simulink model "BalanceSimulink"  (R2023b)
settings: Solver=ode14x  StartTime=0.0  StopTime=100  FixedStep=0.01  MaxStep=0.005  MinStep=0.001  RelTol=1e-3  EnableMultiTasking=on
InitFcn:
  | params_system;
  | RotaryPendulum_SimscapeData;
undefined symbols (not defined in the file or in its folder): k_m, smiData, sp_theta, X, Y, Z
libraries: sm_lib x25, nesl_utility x9, fl_lib x8, simulink x5, ee_lib x1, sdl_lib x1, rllib x1
settings Model: SimulationMode=accelerator  ExtModeTrigDuration=10000  Creator=hongquan  LastModifiedBy=hongquan
settings SolverCC: AlgebraicLoopSolver=TrustRegion  PositivePriorityOrder=on
settings DataIOCC: ReturnWorkspaceOutputs=off
settings DebuggingCC: UnconnectedInputMsg=warning  UnconnectedOutputMsg=warning  UnconnectedLineMsg=warning  ArithmeticOperatorsInVariantConditions=warning
settings ModelReferenceCC: EnableRefExpFcnMdlSchedulingChecks=on
settings SFSimCC: SimUseLocalCustomCode=off  CustomCodeUndefinedFunction=UseInterfaceOnly  SimTargetLang=C++
settings RTWCC: RTWUseLocalCustomCode=off
settings CodeAppCC: StateflowObjectComments=on
settings ConfigComp: CovMetricSettings=dswe

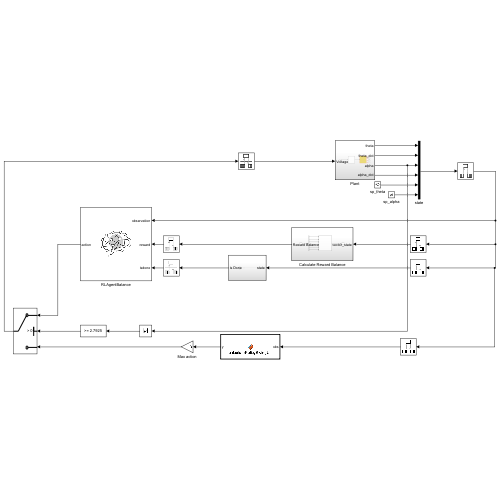
[thumbnail: Simulink's stored preview of the top-level diagram]
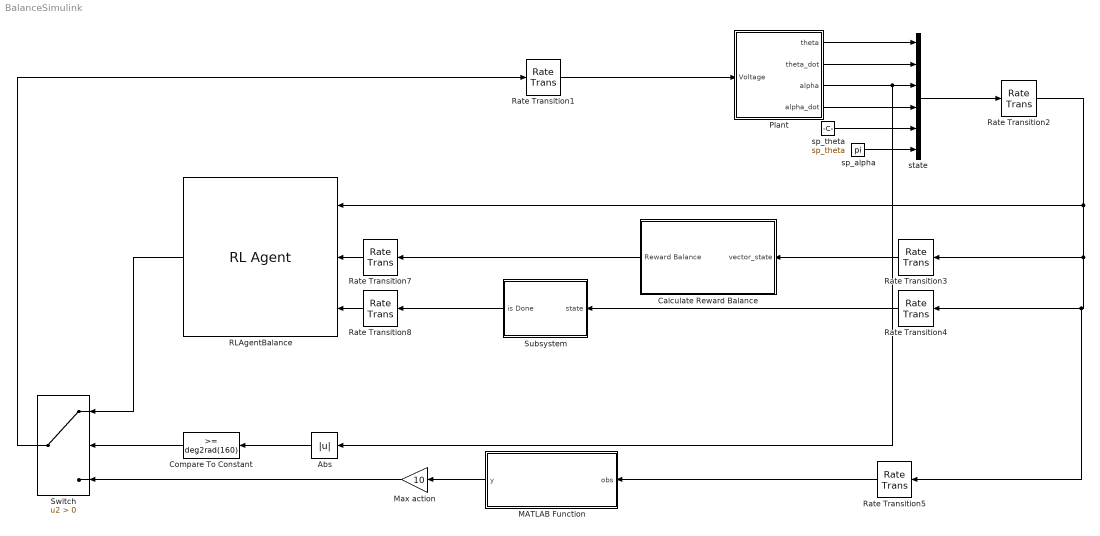
== system BalanceSimulink ==
  Abs : Abs  SaturateOnIntegerOverflow=off
  Calculate Reward Balance : Subsystem
  Compare To Constant : simulink/Logic and Bit Operations/Compare To Constant  relop=>=  const=deg2rad(160)  OutDataTypeStr=boolean
  MATLAB Function : MATLAB Function  TreatAsAtomicUnit=on
  Max action : Gain  Gain=10
  Plant : Subsystem
  RLAgentBalance : rllib/RL Agent  Agent=agent_b  ExternalActionAsInput=off  ProvideLastAction=off  ProvideCumRwd=off  TreatAsDirectFeedthrough=on  UseStrictObservationDataTypes=off
  Rate Transition{1..5,7..8} (7 alike) : RateTransition
  Subsystem : Subsystem
  Switch : Switch  Criteria=u2 > Threshold  SaturateOnIntegerOverflow=off  InputSameDT=off
  sp_alpha : Constant  Value=pi
  sp_theta : Constant  Value=sp_theta
  state : Mux  Inputs=6
  wires:
  state/1 -> Rate Transition2/1
  Plant/1(theta) -> state/1
  Plant/2(theta_dot) -> state/2
  Plant/4(alpha_dot) -> state/4
  sp_theta/1 -> state/5
  sp_alpha/1 -> state/6
  Rate Transition1/1 -> Plant/1(Voltage)
  RLAgentBalance/1 -> Switch/1
  Rate Transition3/1 -> Calculate Reward Balance/1(vector_state)
  Rate Transition8/1 -> RLAgentBalance/3
  Calculate Reward Balance/1(Reward Balance) -> Rate Transition7/1
  Rate Transition7/1 -> RLAgentBalance/2
  Subsystem/1(is Done) -> Rate Transition8/1
  Plant/3(alpha) -> Abs/1, state/3
  Rate Transition4/1 -> Subsystem/1(state)
  Abs/1 -> Compare To Constant/1
  Switch/1 -> Rate Transition1/1
  Rate Transition5/1 -> MATLAB Function/1(obs)
  Compare To Constant/1 -> Switch/2
  Rate Transition2/1 -> Rate Transition5/1, Rate Transition4/1, Rate Transition3/1, RLAgentBalance/1
  MATLAB Function/1(y) -> Max action/1
  Max action/1 -> Switch/3

== system BalanceSimulink/Calculate Reward Balance ==
  vector_state : Inport
  Demux1 : Demux  Outputs=6
  Reward : Subsystem
  Reward Balance : Outport
  wires:
  Demux1/4 -> Reward/4(alpha_dot)
  Demux1/5 -> Reward/5(setpoint_theta)
  Reward/1(reward) -> Reward Balance/1
  Demux1/3 -> Reward/3(alpha)
  Demux1/1 -> Reward/1(theta)
  vector_state/1 -> Demux1/1
  Demux1/2 -> Reward/2(theta_dot)
  Demux1/6 -> Reward/6(setpoint_alpha)

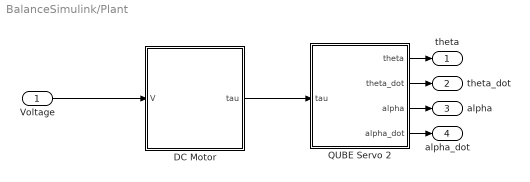
== system BalanceSimulink/Plant ==
  Voltage : Inport
  DC Motor : Subsystem
  QUBE Servo 2 : Subsystem
  theta : Outport
  theta_dot : Outport  Port=2
  alpha : Outport  Port=3
  alpha_dot : Outport  Port=4
  wires:
  QUBE Servo 2/3(" alpha") -> alpha/1
  QUBE Servo 2/2(theta_dot) -> theta_dot/1
  QUBE Servo 2/1(" theta") -> theta/1
  QUBE Servo 2/4(" alpha_dot") -> alpha_dot/1
  Voltage/1 -> DC Motor/1(V)
  DC Motor/1(tau) -> QUBE Servo 2/1(tau)

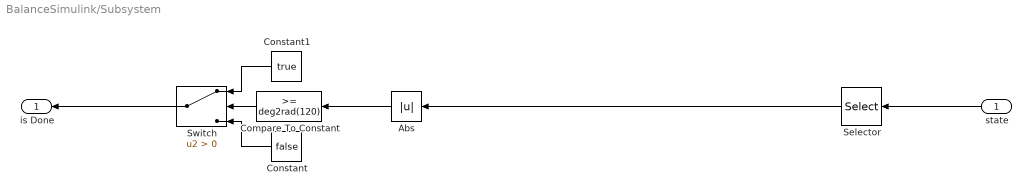
== system BalanceSimulink/Subsystem ==
  state : Inport
  Abs : Abs  SaturateOnIntegerOverflow=off
  Compare To Constant : simulink/Logic and Bit Operations/Compare To Constant  relop=>=  const=deg2rad(120)  OutDataTypeStr=boolean
  Constant : Constant  Value=false
  Constant1 : Constant  Value=true
  Selector : Selector  InputPortWidth=6  IndexOptions=Index vector (dialog)  Indices=[1]  OutputSizes=1
  Switch : Switch  Criteria=u2 > Threshold  SaturateOnIntegerOverflow=off  InputSameDT=off
  is Done : Outport
  wires:
  Constant1/1 -> Switch/1
  Compare To Constant/1 -> Switch/2
  Abs/1 -> Compare To Constant/1
  Constant/1 -> Switch/3
  state/1 -> Selector/1
  Selector/1 -> Abs/1
  Switch/1 -> is Done/1

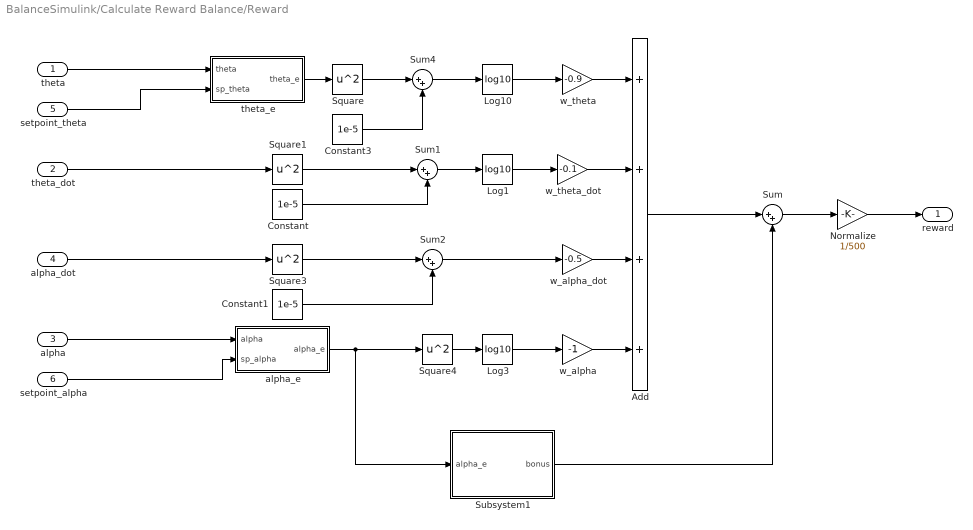
== system BalanceSimulink/Calculate Reward Balance/Reward ==
  theta : Inport
  theta_dot : Inport  Port=2
  alpha : Inport  Port=3
  alpha_dot : Inport  Port=4
  setpoint_theta : Inport  Port=5
  setpoint_alpha : Inport  Port=6
  Add : Sum  Inputs=++++
  Constant : Constant  Value=1e-5
  Constant1 : Constant  Value=1e-5
  Constant3 : Constant  Value=1e-5
  Log1 : Math  Operator=log10
  Log10 : Math  Operator=log10
  Log3 : Math  Operator=log10
  Normalize : Gain  Gain=1/500
  Square{,1,3..4} (4 alike) : Math  Operator=square
  Subsystem1 : Subsystem
  Sum{,1..2,4} (4 alike) : Sum  Inputs=|++
  alpha_e : Subsystem
  theta_e : Subsystem
  w_alpha : Gain  Gain=-1
  w_alpha_dot : Gain  Gain=-0.5
  w_theta : Gain  Gain=-0.9
  w_theta_dot : Gain  Gain=-0.1
  reward : Outport
  wires:
  Log3/1 -> w_alpha/1
  Log1/1 -> w_theta_dot/1
  Log10/1 -> w_theta/1
  theta_e/1(theta_e) -> Square/1
  w_theta/1 -> Add/1
  setpoint_theta/1 -> theta_e/2(sp_theta)
  w_theta_dot/1 -> Add/2
  setpoint_alpha/1 -> alpha_e/2(sp_alpha)
  alpha/1 -> alpha_e/1(alpha)
  theta/1 -> theta_e/1(theta)
  w_alpha_dot/1 -> Add/3
  w_alpha/1 -> Add/4
  Add/1 -> Sum/1
  Sum/1 -> Normalize/1
  Subsystem1/1(bonus) -> Sum/2
  Normalize/1 -> reward/1
  Square4/1 -> Log3/1
  theta_dot/1 -> Square1/1
  alpha_dot/1 -> Square3/1
  Constant1/1 -> Sum2/2
  Constant/1 -> Sum1/2
  Square1/1 -> Sum1/1
  Sum1/1 -> Log1/1
  Square3/1 -> Sum2/1
  alpha_e/1(alpha_e) -> Square4/1, Subsystem1/1(alpha_e)
  Constant3/1 -> Sum4/2
  Square/1 -> Sum4/1
  Sum4/1 -> Log10/1
  Sum2/1 -> w_alpha_dot/1

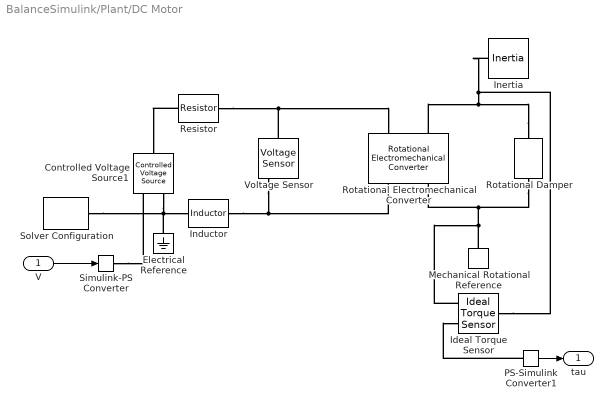
== system BalanceSimulink/Plant/DC Motor ==
  V : Inport
  Controlled Voltage Source1 : fl_lib/Electrical/Electrical Sources/Controlled Voltage Source
  Electrical Reference : fl_lib/Electrical/Electrical Elements/Electrical Reference
  Ideal Torque Sensor : fl_lib/Mechanical/Mechanical Sensors/Ideal Torque Sensor
  Inductor : ee_lib/Passive/Inductor  l=L_m H  enable_L_tol=ee.enum.toleranceApplication.none  L_tol=20  tol_distribution=ee.enum.toleranceDistribution.uniform  nSigma=4  r=R_m Ohm  g=1e-9 1/Ohm  enable_operating_limits=ee.enum.enable.no  operating_limit_action=ee.enum.passive.reportOpLim.warn  max_working_current=1 A  power_rating=1 W  enable_faults=ee.enum.enable.no  fault_action=simscape.enum.assert.action.none  lambdaPercent=50  k_faulted=0.9999  turnsShort=ee.enum.passive.inductor.turnsShortOption.no  openCct=ee.enum.enable.no  groundShort=ee.enum.passive.inductor.groundShortOption.no  groundShortG=0 1/Ohm  tau_fault=1e-3 s  fault_trigger=ee.enum.faults.faultTrigger.temporal  t_fault=1 s  max_permissible_voltage=100 V  n_fail_on_voltage=1  max_permissible_current=1 A  t_fail_on_current=1 s  i_L_specify=off  i_L_priority=High  i_L=0 A  i_L_nominal_specify=off  i_L_nominal_unit=A  i_L_nominal_value=1
  Inertia : fl_lib/Mechanical/Rotational Elements/Inertia  inertia=J_m kg*m^2  num_ports=foundation.enum.numPorts2.one  w_specify=off  w_priority=High  w=0 rad/s  w_nominal_specify=on  w_nominal_unit=rad/s  w_nominal_value=omega_nom  t_specify=off  t_priority=None  t=0 N*m  t_nominal_specify=on  t_nominal_unit=N*m  t_nominal_value=tau_nom
  Mechanical Rotational Reference : fl_lib/Mechanical/Rotational Elements/Mechanical Rotational Reference
  PS-Simulink Converter1 : nesl_utility/PS-Simulink Converter  PhysicalDomain=network_engine_domain  SubClassName=ps_output  LeftPortType=input  RightPortType=output  PseudoPeriodic=off  Frequencies=[]  VectorFormat=inherit  Unit=inherit  AffineConversion=off
  Resistor : fl_lib/Electrical/Electrical Elements/Resistor  R=8.4 Ohm  i_specify=off  i_priority=None  i=0 A  i_nominal_specify=on  i_nominal_unit=mA  i_nominal_value=22  v_specify=off  v_priority=None  v=0 V  v_nominal_specify=on  v_nominal_unit=V  v_nominal_value=18
  Rotational Electromechanical Converter : fl_lib/Electrical/Electrical Elements/Rotational Electromechanical Converter  K=k_m V*s/rad  i_specify=off  i_priority=None  i=0 A  i_nominal_specify=on  i_nominal_unit=mA  i_nominal_value=I_nom  v_specify=off  v_priority=None  v=0 V  v_nominal_specify=on  v_nominal_unit=V  v_nominal_value=V_nom  t_specify=off  t_priority=None  t=0 N*m  t_nominal_specify=on  t_nominal_unit=N*m  t_nominal_value=tau_nom  w_specify=off  w_priority=None  w=0 rad/s  w_nominal_specify=on  w_nominal_unit=rad/s  w_nominal_value=omega_nom
  Rotational Damper : sdl_lib/Couplings & Drives/Springs & Dampers/Rotational Damper  D=0.2 N*m*s/rad  enable_faults=simscape.enum.onoff.off  b_fault=100 N*m*s/rad  temporal_fault=simscape.enum.onoff.off  fault_time=5 s  shock_fault=simscape.enum.onoff.off  acceleration_limit=100 rad/s^2  shock_limit=1  report_fault=simscape.enum.assert.action.none  thermal_port=simscape.enum.thermaleffects.omit  thermal_mass=50 kJ/K  temperature_specify=off  temperature_priority=High  temperature=300 K  temperature_nominal_specify=off  temperature_nominal_unit=K  temperature_nominal_value=1
  Simulink-PS Converter : nesl_utility/Simulink-PS Converter  PhysicalDomain=network_engine_domain  SubClassName=ps_input  LeftPortType=input  RightPortType=output  PseudoPeriodic=off  Frequencies=[]  NoiseDistribution=none  NoiseParameters=[]  Unit=1  AffineConversion=off  FilteringAndDerivatives=zero  SimscapeFilterOrder=1  InputFilterTimeConstant=0.01  UdotUserProvided=0
  Solver Configuration : nesl_utility/Solver Configuration  PhysicalDomain=network_engine_domain  SubClassName=solver  LeftPortType=input  RightPortType=generic  Tones=[]  Harmonics=[]  SimulateNoise=off  Profile=off  UseLocalSampling=off  EnableSwitchedLinearOptims=on  FrequencyDomain=off  UseCCode=off  RelTol=0.001  AbsTol=0.001  MinStep=1e-09  ToWorkspace=off  RevertToSquareIcSolve=off  NumHomotopyIterations=100  PhasorMode=off  PhasorModeNumHarmonics=1  ConsistencySolver=NEWTON_XTOL_AFTER_FTOL  IndexReductionMethod=DerivativeReplacement  DoDC=off  ResidualTolerance=1e-09  ConsistencyTolSource=GLOBAL  ConsistencyAbsTol=0.001  ConsistencyRelTol=0.001  ConsistencyTolFactor=0.001  UseLocalSolver=off  LocalSolverChoice=NE_BACKWARD_EULER_ADVANCER  ResolveIndetEquations=on  FunctionEvalNumThread=1  LocalSolverSampleTime=0.001  DoFixedCost=off  MaxNonlinIter=3  MaxModeIter=2  ComputeImpulses=off  ImpulseIterations=2  LinearAlgebra=auto  LinearAlgebraNumThread=0  EquationFormulation=NE_TIME_EF  DelaysMemoryBudget=1024  AutomaticFiltering=off  FilteringTimeConstant=0.001  PartitionStorageMethod=AS_NEEDED  PartitionMemoryBudget=1024  PartitionMethod=ROBUST  MultibodyUseLocalSolver=off  MultibodyLocalSolverChoice=ODE1  MultibodyLocalSolverSampleTime=0.001
  Voltage Sensor : fl_lib/Electrical/Electrical Sensors/Voltage Sensor
  tau : Outport
  wires:
  PS-Simulink Converter1/1 -> tau/1
  V/1 -> Simulink-PS Converter/1
  connections:
  Resistor/LConn1 -- Controlled Voltage Source1/LConn1
  Simulink-PS Converter/RConn1 -- Controlled Voltage Source1/RConn1
  Resistor/RConn1 -- Rotational Electromechanical Converter/LConn1 -- Voltage Sensor/LConn1
  PS-Simulink Converter1/LConn1 -- Ideal Torque Sensor/RConn2
  Rotational Electromechanical Converter/RConn2 -- Rotational Damper/RConn1 -- Mechanical Rotational Reference/LConn1 -- Ideal Torque Sensor/RConn1
  Voltage Sensor/RConn2 -- Inductor/RConn1 -- Rotational Electromechanical Converter/RConn1
  Rotational Damper/LConn1 -- Rotational Electromechanical Converter/LConn2 -- Inertia/LConn1 -- Ideal Torque Sensor/LConn1
  Solver Configuration/RConn1 -- Controlled Voltage Source1/RConn2 -- Electrical Reference/LConn1 -- Inductor/LConn1

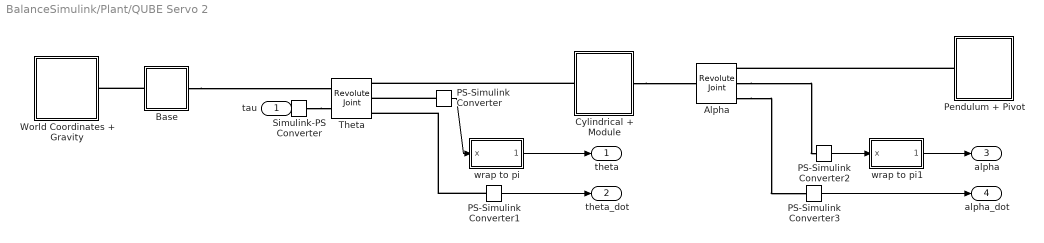
== system BalanceSimulink/Plant/QUBE Servo 2 ==
  tau : Inport
  Alpha : sm_lib/Joints/Revolute Joint  JointMode=Normal  SenseConstraintForce=off  SenseConstraintForceX=off  SenseConstraintForceY=off  SenseConstraintForceZ=off  SenseConstraintTorque=off  SenseConstraintTorqueX=off  SenseConstraintTorqueY=off  SenseConstraintTorqueZ=off  SenseTotalForce=off  SenseTotalForceX=off  SenseTotalForceY=off  SenseTotalForceZ=off  SenseTotalTorque=off  SenseTotalTorqueX=off  SenseTotalTorqueY=off  SenseTotalTorqueZ=off  CompositeWrenchDir=FollowerOnBase  CompositeWrenchFrame=BaseFrame  EquilibriumPosition=0  EquilibriumPositionUnits=deg  SpringStiffness=0  SpringStiffnessUnits=N*m/deg  DampingCoefficient=1e-7  DampingCoefficientUnits=N*m/(deg/s)  TorqueActuationMode=NoTorque  MotionActuationMode=ComputedMotion  SensePosition=on  SenseVelocity=on  SenseAcceleration=off  SenseTorqueForce=off  SenseLowerLimitTorqueForce=off  SenseUpperLimitTorqueForce=off  LowerLimitSpecify=off  LowerLimitBound=-90  LowerLimitBoundUnits=deg  LowerLimitStiffness=1e4  LowerLimitStiffnessUnits=N*m/deg  LowerLimitDamping=10  LowerLimitDampingUnits=N*m/(deg/s)  LowerLimitTransitionRegionWidth=0.1  LowerLimitTransitionRegionWidthUnits=deg  UpperLimitSpecify=off  UpperLimitBound=90  UpperLimitBoundUnits=deg  UpperLimitStiffness=1e4  UpperLimitStiffnessUnits=N*m/deg  UpperLimitDamping=10  UpperLimitDampingUnits=N*m/(deg/s)  UpperLimitTransitionRegionWidth=0.1  UpperLimitTransitionRegionWidthUnits=deg  PositionTargetSpecify=off  PositionTargetPriority=High  PositionTargetValue=pi  PositionTargetValueUnits=rad  VelocityTargetSpecify=off  VelocityTargetPriority=High  VelocityTargetValue=0  VelocityTargetValueUnits=deg/s
  Base : Subsystem
  Cylindrical + Module : Subsystem
  PS-Simulink Converter{,1..3} (4 alike) : nesl_utility/PS-Simulink Converter  PhysicalDomain=network_engine_domain  SubClassName=ps_output  LeftPortType=input  RightPortType=output  PseudoPeriodic=off  Frequencies=[]  VectorFormat=inherit  Unit=inherit  AffineConversion=off
  Pendulum + Pivot : Subsystem
  Simulink-PS Converter : nesl_utility/Simulink-PS Converter  PhysicalDomain=network_engine_domain  SubClassName=ps_input  LeftPortType=input  RightPortType=output  PseudoPeriodic=off  Frequencies=[]  NoiseDistribution=none  NoiseParameters=[]  Unit=N*m  AffineConversion=off  FilteringAndDerivatives=zero  SimscapeFilterOrder=1  InputFilterTimeConstant=0.01  UdotUserProvided=0
  Theta : sm_lib/Joints/Revolute Joint  JointMode=Normal  SenseConstraintForce=off  SenseConstraintForceX=off  SenseConstraintForceY=off  SenseConstraintForceZ=off  SenseConstraintTorque=off  SenseConstraintTorqueX=off  SenseConstraintTorqueY=off  SenseConstraintTorqueZ=off  SenseTotalForce=off  SenseTotalForceX=off  SenseTotalForceY=off  SenseTotalForceZ=off  SenseTotalTorque=off  SenseTotalTorqueX=off  SenseTotalTorqueY=off  SenseTotalTorqueZ=off  CompositeWrenchDir=FollowerOnBase  CompositeWrenchFrame=BaseFrame  EquilibriumPosition=0  EquilibriumPositionUnits=rad  SpringStiffness=0  SpringStiffnessUnits=N*m/rad  DampingCoefficient=1e-7  DampingCoefficientUnits=N*m/(deg/s)  TorqueActuationMode=InputTorque  MotionActuationMode=ComputedMotion  SensePosition=on  SenseVelocity=on  SenseAcceleration=off  SenseTorqueForce=off  SenseLowerLimitTorqueForce=off  SenseUpperLimitTorqueForce=off  LowerLimitSpecify=off  LowerLimitBound=-90  LowerLimitBoundUnits=deg  LowerLimitStiffness=1e4  LowerLimitStiffnessUnits=N*m/deg  LowerLimitDamping=10  LowerLimitDampingUnits=N*m/(deg/s)  LowerLimitTransitionRegionWidth=0.1  LowerLimitTransitionRegionWidthUnits=deg  UpperLimitSpecify=off  UpperLimitBound=90  UpperLimitBoundUnits=deg  UpperLimitStiffness=1e4  UpperLimitStiffnessUnits=N*m/deg  UpperLimitDamping=10  UpperLimitDampingUnits=N*m/(deg/s)  UpperLimitTransitionRegionWidth=0.1  UpperLimitTransitionRegionWidthUnits=deg  PositionTargetSpecify=off  PositionTargetPriority=Low  PositionTargetValue=theta_init  PositionTargetValueUnits=deg  VelocityTargetSpecify=off  VelocityTargetPriority=High  VelocityTargetValue=0  VelocityTargetValueUnits=rad/s
  World Coordinates + Gravity : Subsystem
  wrap to pi : Subsystem
  wrap to pi1 : Subsystem
  " theta" : Outport
  theta_dot : Outport  Port=2
  " alpha" : Outport  Port=3
  " alpha_dot" : Outport  Port=4
  wires:
  PS-Simulink Converter/1 -> wrap to pi/1(x)
  PS-Simulink Converter2/1 -> wrap to pi1/1(x)
  PS-Simulink Converter3/1 -> " alpha_dot"/1
  PS-Simulink Converter1/1 -> theta_dot/1
  wrap to pi/1(x_wrapped) -> " theta"/1
  wrap to pi1/1(x_wrapped) -> " alpha"/1
  tau/1 -> Simulink-PS Converter/1
  connections:
  Alpha/RConn3 -- PS-Simulink Converter3/LConn1
  Alpha/RConn2 -- PS-Simulink Converter2/LConn1
  PS-Simulink Converter1/LConn1 -- Theta/RConn3
  PS-Simulink Converter/LConn1 -- Theta/RConn2
  Simulink-PS Converter/RConn1 -- Theta/LConn2
  Cylindrical + Module/LConn1 -- Theta/RConn1
  Base/LConn1 -- World Coordinates + Gravity/RConn1
  Pendulum + Pivot/LConn1 -- Alpha/RConn1
  Cylindrical + Module/RConn1 -- Alpha/LConn1
  Base/RConn1 -- Theta/LConn1

== system BalanceSimulink/Calculate Reward Balance/Reward/Subsystem1 ==
  alpha_e : Inport
  Abs : Abs  SaturateOnIntegerOverflow=off
  Stay at pi : Subsystem
  bonus : Outport
  wires:
  alpha_e/1 -> Abs/1
  Abs/1 -> Stay at pi/1(abs(alpha_e))
  Stay at pi/1(bonus) -> bonus/1

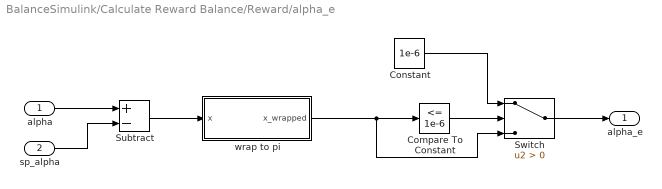
== system BalanceSimulink/Calculate Reward Balance/Reward/alpha_e ==
  alpha : Inport
  sp_alpha : Inport  Port=2
  Compare To Constant : simulink/Logic and Bit Operations/Compare To Constant  relop=<=  const=1e-6  OutDataTypeStr=boolean
  Constant : Constant  Value=1e-6
  Subtract : Sum  Inputs=+-
  Switch : Switch  Criteria=u2 > Threshold  SaturateOnIntegerOverflow=off  InputSameDT=off
  wrap to pi : Subsystem
  alpha_e : Outport
  wires:
  wrap to pi/1(x_wrapped) -> Switch/3, Compare To Constant/1
  Constant/1 -> Switch/1
  Switch/1 -> alpha_e/1
  Compare To Constant/1 -> Switch/2
  Subtract/1 -> wrap to pi/1(x)
  sp_alpha/1 -> Subtract/2
  alpha/1 -> Subtract/1

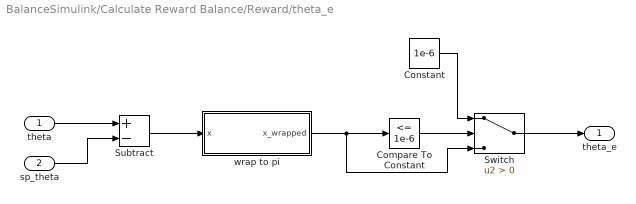
== system BalanceSimulink/Calculate Reward Balance/Reward/theta_e ==
  theta : Inport
  sp_theta : Inport  Port=2
  Compare To Constant : simulink/Logic and Bit Operations/Compare To Constant  relop=<=  const=1e-6  OutDataTypeStr=boolean
  Constant : Constant  Value=1e-6
  Subtract : Sum  Inputs=+-
  Switch : Switch  Criteria=u2 > Threshold  SaturateOnIntegerOverflow=off  InputSameDT=off
  wrap to pi : Subsystem
  theta_e : Outport
  wires:
  Subtract/1 -> wrap to pi/1(x)
  sp_theta/1 -> Subtract/2
  theta/1 -> Subtract/1
  wrap to pi/1(x_wrapped) -> Switch/3, Compare To Constant/1
  Compare To Constant/1 -> Switch/2
  Switch/1 -> theta_e/1
  Constant/1 -> Switch/1

== system BalanceSimulink/Plant/QUBE Servo 2/Base ==
  ReferenceFrame : sm_lib/Frames and Transforms/Reference Frame
  Solid : sm_lib/Body Elements/File Solid  ExtGeomFileName=Base_Default_sldprt.STEP  UnitType=FromFile  ExtGeomFileUnits=m  StepReaderType=HEX  ExportConvexHullGeometry=off  InertiaType=Custom  Mass=smiData.Solid(1).mass  MassUnits=kg  CenterOfMass=smiData.Solid(1).CoM  CenterOfMassUnits=mm  MomentsOfInertia=smiData.Solid(1).MoI  MomentsOfInertiaUnits=kg*mm^2  ProductsOfInertia=smiData.Solid(1).PoI  ProductsOfInertiaUnits=kg*mm^2  BasedOnType=DensityFromFile  Density=1000  DensityUnits=kg/m^3  DoExposeReferenceFrame=on  SerializedFrames=<Frames/>  GraphicType=FromGeometry  MarkerShape=Sphere  MarkerSize=10  GraphicVisPropType=SimpleVisualProperties  GraphicDiffuseColor=[0.6 0.6 0.6]  GraphicSpecularColor=[0.5 0.5 0.5 1.0]  GraphicAmbientColor=[0.15 0.15 0.15 1.0]  GraphicEmissiveColor=[0.0 0.0 0.0 1.0]  GraphicShininess=75  GraphicOpacity=smiData.Solid(1).opacity
  Transform : sm_lib/Frames and Transforms/Rigid Transform  TranslationMethod=Cartesian  TranslationStandardOffset=0  TranslationStandardOffsetUnits=m  TranslationStandardAxis=+Z  TranslationCartesianOffset=smiData.RigidTransform(5).translation  TranslationCartesianOffsetUnits=mm  TranslationROffset=0  TranslationROffsetUnits=m  TranslationZOffset=0  TranslationZOffsetUnits=m  TranslationThetaOffset=0  TranslationThetaOffsetUnits=deg  RotationMethod=ArbitraryAxis  RotationAngleUnits=rad  RotationStandardAxis=+Z  RotationAngle=smiData.RigidTransform(5).angle  RotationArbitraryAxis=smiData.RigidTransform(5).axis  FollAlignAxisA=+X  BaseAlignAxisA=+Y  FollAlignAxisB=+Y  BaseAlignAxisB=+Z  RotationSequenceAxes=FollowerAxes  RotationSequence=XYX  RotationSequenceAngles=[0 0 0]  RotationSequenceAnglesUnits=deg  RotationMatrix=[1 0 0; 0 1 0; 0 0 1]  Quaternion=[1 0 0 0]
  Transform1 : sm_lib/Frames and Transforms/Rigid Transform  TranslationMethod=Cartesian  TranslationStandardOffset=0  TranslationStandardOffsetUnits=m  TranslationStandardAxis=+Z  TranslationCartesianOffset=smiData.RigidTransform(7).translation  TranslationCartesianOffsetUnits=mm  TranslationROffset=0  TranslationROffsetUnits=m  TranslationZOffset=0  TranslationZOffsetUnits=m  TranslationThetaOffset=0  TranslationThetaOffsetUnits=deg  RotationMethod=ArbitraryAxis  RotationAngleUnits=rad  RotationStandardAxis=+Z  RotationAngle=smiData.RigidTransform(7).angle  RotationArbitraryAxis=smiData.RigidTransform(7).axis  FollAlignAxisA=+X  BaseAlignAxisA=+Y  FollAlignAxisB=+Y  BaseAlignAxisB=+Z  RotationSequenceAxes=FollowerAxes  RotationSequence=XYX  RotationSequenceAngles=[0 0 0]  RotationSequenceAnglesUnits=deg  RotationMatrix=[1 0 0; 0 1 0; 0 0 1]  Quaternion=[1 0 0 0]
  F : PMIOPort  Side=Left
  F1 : PMIOPort  Port=2  Side=Right
  connections:
  Transform1/RConn1 -- F1/RConn1
  Transform/RConn1 -- F/RConn1
  Transform1/LConn1 -- Transform/LConn1 -- ReferenceFrame/RConn1 -- Solid/RConn1

== system BalanceSimulink/Plant/QUBE Servo 2/Cylindrical + Module ==
  Circle : Subsystem
  Module : Subsystem
  F : PMIOPort  Side=Right
  F1 : PMIOPort  Port=2  Side=Left
  connections:
  Circle/LConn2 -- F1/RConn1
  Module/RConn1 -- F/RConn1
  Circle/LConn1 -- Module/LConn1

== system BalanceSimulink/Plant/QUBE Servo 2/Pendulum + Pivot ==
  Pendulum : Subsystem
  Pivot : Subsystem
  F : PMIOPort  Side=Left
  connections:
  Pivot/LConn2 -- F/RConn1
  Pendulum/LConn1 -- Pivot/LConn1

== system BalanceSimulink/Plant/QUBE Servo 2/World Coordinates + Gravity ==
  MechanismConfiguration : sm_lib/Utilities/Mechanism Configuration  UniformGravity=Constant  GravityVector=[0 0 -9.78]  GravityVectorUnits=m/s^2  LinearizationDelta=0.001  JointModeTransitionNonlinearIterations=2
  Solver Configuration : nesl_utility/Solver Configuration  PhysicalDomain=network_engine_domain  SubClassName=solver  LeftPortType=input  RightPortType=generic  Tones=[]  Harmonics=[]  SimulateNoise=off  Profile=off  UseLocalSampling=off  EnableSwitchedLinearOptims=on  FrequencyDomain=off  UseCCode=off  RelTol=0.001  AbsTol=0.001  MinStep=1e-09  ToWorkspace=off  RevertToSquareIcSolve=off  NumHomotopyIterations=100  PhasorMode=off  PhasorModeNumHarmonics=1  ConsistencySolver=NEWTON_XTOL_AFTER_FTOL  IndexReductionMethod=DerivativeReplacement  DoDC=off  ResidualTolerance=1e-09  ConsistencyTolSource=GLOBAL  ConsistencyAbsTol=0.001  ConsistencyRelTol=0.001  ConsistencyTolFactor=0.001  UseLocalSolver=off  LocalSolverChoice=NE_BACKWARD_EULER_ADVANCER  ResolveIndetEquations=on  FunctionEvalNumThread=1  LocalSolverSampleTime=0.001  DoFixedCost=off  MaxNonlinIter=3  MaxModeIter=2  ComputeImpulses=off  ImpulseIterations=2  LinearAlgebra=auto  LinearAlgebraNumThread=0  EquationFormulation=NE_TIME_EF  DelaysMemoryBudget=1024  AutomaticFiltering=off  FilteringTimeConstant=0.001  PartitionStorageMethod=AS_NEEDED  PartitionMemoryBudget=1024  PartitionMethod=ROBUST  MultibodyUseLocalSolver=off  MultibodyLocalSolverChoice=ODE1  MultibodyLocalSolverSampleTime=0.001
  Transform : sm_lib/Frames and Transforms/Rigid Transform  TranslationMethod=Cartesian  TranslationStandardOffset=0  TranslationStandardOffsetUnits=m  TranslationStandardAxis=+Z  TranslationCartesianOffset=smiData.RigidTransform(6).translation  TranslationCartesianOffsetUnits=mm  TranslationROffset=0  TranslationROffsetUnits=m  TranslationZOffset=0  TranslationZOffsetUnits=m  TranslationThetaOffset=0  TranslationThetaOffsetUnits=deg  RotationMethod=ArbitraryAxis  RotationAngleUnits=rad  RotationStandardAxis=+Z  RotationAngle=smiData.RigidTransform(6).angle  RotationArbitraryAxis=smiData.RigidTransform(6).axis  FollAlignAxisA=+X  BaseAlignAxisA=+Y  FollAlignAxisB=+Y  BaseAlignAxisB=+Z  RotationSequenceAxes=FollowerAxes  RotationSequence=XYX  RotationSequenceAngles=[0 0 0]  RotationSequenceAnglesUnits=deg  RotationMatrix=[1 0 0; 0 1 0; 0 0 1]  Quaternion=[1 0 0 0]
  World : sm_lib/Frames and Transforms/World Frame
  Conn1 : PMIOPort  Side=Right
  connections:
  Conn1/RConn1 -- Transform/RConn1
  World/RConn1 -- Solver Configuration/RConn1 -- MechanismConfiguration/RConn1 -- Transform/LConn1

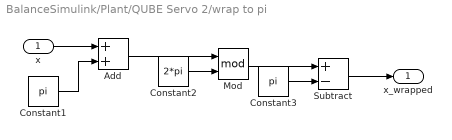
== system BalanceSimulink/Plant/QUBE Servo 2/wrap to pi ==
  x : Inport
  Add : Sum
  Constant1 : Constant  Value=pi
  Constant2 : Constant  Value=2*pi
  Constant3 : Constant  Value=pi
  Mod : Math  Operator=mod
  Subtract : Sum  Inputs=+-
  x_wrapped : Outport
  wires:
  Mod/1 -> Subtract/1
  Constant3/1 -> Subtract/2
  Subtract/1 -> x_wrapped/1
  Add/1 -> Mod/1
  x/1 -> Add/1
  Constant1/1 -> Add/2
  Constant2/1 -> Mod/2

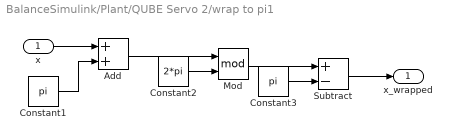
== system BalanceSimulink/Plant/QUBE Servo 2/wrap to pi1 ==
  x : Inport
  Add : Sum
  Constant1 : Constant  Value=pi
  Constant2 : Constant  Value=2*pi
  Constant3 : Constant  Value=pi
  Mod : Math  Operator=mod
  Subtract : Sum  Inputs=+-
  x_wrapped : Outport
  wires:
  Mod/1 -> Subtract/1
  Constant3/1 -> Subtract/2
  Subtract/1 -> x_wrapped/1
  Add/1 -> Mod/1
  x/1 -> Add/1
  Constant1/1 -> Add/2
  Constant2/1 -> Mod/2

== system BalanceSimulink/Calculate Reward Balance/Reward/Subsystem1/Stay at pi ==
  abs(alpha_e) : Inport
  Compare To Deg2Rad(2) : simulink/Logic and Bit Operations/Compare To Constant  relop=<=  const=deg2rad(2)  OutDataTypeStr=boolean
  Constant : Constant  Value=200
  Constant1 : Constant  Value=0
  Switch : Switch  Criteria=u2 > Threshold  SaturateOnIntegerOverflow=off  InputSameDT=off
  bonus : Outport
  wires:
  Constant1/1 -> Switch/3
  Compare To Deg2Rad(2)/1 -> Switch/2
  Constant/1 -> Switch/1
  abs(alpha_e)/1 -> Compare To Deg2Rad(2)/1
  Switch/1 -> bonus/1

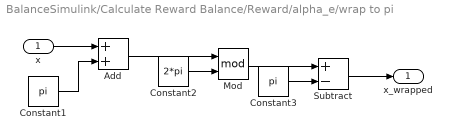
== system BalanceSimulink/Calculate Reward Balance/Reward/alpha_e/wrap to pi ==
  x : Inport
  Add : Sum
  Constant1 : Constant  Value=pi
  Constant2 : Constant  Value=2*pi
  Constant3 : Constant  Value=pi
  Mod : Math  Operator=mod
  Subtract : Sum  Inputs=+-
  x_wrapped : Outport
  wires:
  Constant2/1 -> Mod/2
  Constant1/1 -> Add/2
  x/1 -> Add/1
  Add/1 -> Mod/1
  Subtract/1 -> x_wrapped/1
  Constant3/1 -> Subtract/2
  Mod/1 -> Subtract/1

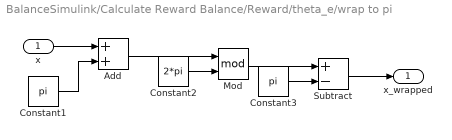
== system BalanceSimulink/Calculate Reward Balance/Reward/theta_e/wrap to pi ==
  x : Inport
  Add : Sum
  Constant1 : Constant  Value=pi
  Constant2 : Constant  Value=2*pi
  Constant3 : Constant  Value=pi
  Mod : Math  Operator=mod
  Subtract : Sum  Inputs=+-
  x_wrapped : Outport
  wires:
  Constant2/1 -> Mod/2
  Constant1/1 -> Add/2
  x/1 -> Add/1
  Add/1 -> Mod/1
  Subtract/1 -> x_wrapped/1
  Constant3/1 -> Subtract/2
  Mod/1 -> Subtract/1

== system BalanceSimulink/Plant/QUBE Servo 2/Cylindrical + Module/Circle ==
  ReferenceFrame : sm_lib/Frames and Transforms/Reference Frame
  Solid : sm_lib/Body Elements/File Solid  ExtGeomFileName=Circle_Default_sldprt.STEP  UnitType=FromFile  ExtGeomFileUnits=m  StepReaderType=HEX  ExportConvexHullGeometry=off  InertiaType=Custom  Mass=smiData.Solid(5).mass  MassUnits=kg  CenterOfMass=smiData.Solid(5).CoM  CenterOfMassUnits=mm  MomentsOfInertia=smiData.Solid(5).MoI  MomentsOfInertiaUnits=kg*mm^2  ProductsOfInertia=smiData.Solid(5).PoI  ProductsOfInertiaUnits=kg*mm^2  BasedOnType=DensityFromFile  Density=1000  DensityUnits=kg/m^3  DoExposeReferenceFrame=on  SerializedFrames=<Frames/>  GraphicType=FromGeometry  MarkerShape=Sphere  MarkerSize=10  GraphicVisPropType=SimpleVisualProperties  GraphicDiffuseColor=[1.0 1.0 1.0]  GraphicSpecularColor=[0.5 0.5 0.5 1.0]  GraphicAmbientColor=[0.15 0.15 0.15 1.0]  GraphicEmissiveColor=[0.0 0.0 0.0 1.0]  GraphicShininess=75  GraphicOpacity=smiData.Solid(5).opacity
  Transform : sm_lib/Frames and Transforms/Rigid Transform  TranslationMethod=Cartesian  TranslationStandardOffset=0  TranslationStandardOffsetUnits=m  TranslationStandardAxis=+Z  TranslationCartesianOffset=smiData.RigidTransform(8).translation  TranslationCartesianOffsetUnits=mm  TranslationROffset=0  TranslationROffsetUnits=m  TranslationZOffset=0  TranslationZOffsetUnits=m  TranslationThetaOffset=0  TranslationThetaOffsetUnits=deg  RotationMethod=ArbitraryAxis  RotationAngleUnits=rad  RotationStandardAxis=+Z  RotationAngle=smiData.RigidTransform(8).angle  RotationArbitraryAxis=smiData.RigidTransform(8).axis  FollAlignAxisA=+X  BaseAlignAxisA=+Y  FollAlignAxisB=+Y  BaseAlignAxisB=+Z  RotationSequenceAxes=FollowerAxes  RotationSequence=XYX  RotationSequenceAngles=[0 0 0]  RotationSequenceAnglesUnits=deg  RotationMatrix=[1 0 0; 0 1 0; 0 0 1]  Quaternion=[1 0 0 0]
  Transform1 : sm_lib/Frames and Transforms/Rigid Transform  TranslationMethod=Cartesian  TranslationStandardOffset=0  TranslationStandardOffsetUnits=m  TranslationStandardAxis=+Z  TranslationCartesianOffset=smiData.RigidTransform(9).translation  TranslationCartesianOffsetUnits=mm  TranslationROffset=0  TranslationROffsetUnits=m  TranslationZOffset=0  TranslationZOffsetUnits=m  TranslationThetaOffset=0  TranslationThetaOffsetUnits=deg  RotationMethod=ArbitraryAxis  RotationAngleUnits=rad  RotationStandardAxis=+Z  RotationAngle=smiData.RigidTransform(9).angle  RotationArbitraryAxis=smiData.RigidTransform(9).axis  FollAlignAxisA=+X  BaseAlignAxisA=+Y  FollAlignAxisB=+Y  BaseAlignAxisB=+Z  RotationSequenceAxes=FollowerAxes  RotationSequence=XYX  RotationSequenceAngles=[0 0 0]  RotationSequenceAnglesUnits=deg  RotationMatrix=[1 0 0; 0 1 0; 0 0 1]  Quaternion=[1 0 0 0]
  F1 : PMIOPort  Side=Left
  F : PMIOPort  Port=2  Side=Left
  connections:
  Transform1/RConn1 -- F1/RConn1
  Transform/RConn1 -- F/RConn1
  Transform1/LConn1 -- Transform/LConn1 -- ReferenceFrame/RConn1 -- Solid/RConn1

== system BalanceSimulink/Plant/QUBE Servo 2/Cylindrical + Module/Module ==
  ReferenceFrame : sm_lib/Frames and Transforms/Reference Frame
  Solid : sm_lib/Body Elements/File Solid  ExtGeomFileName=Module_Default_sldprt.STEP  UnitType=FromFile  ExtGeomFileUnits=m  StepReaderType=HEX  ExportConvexHullGeometry=off  InertiaType=Custom  Mass=smiData.Solid(4).mass  MassUnits=kg  CenterOfMass=smiData.Solid(4).CoM  CenterOfMassUnits=mm  MomentsOfInertia=smiData.Solid(4).MoI  MomentsOfInertiaUnits=kg*mm^2  ProductsOfInertia=smiData.Solid(4).PoI  ProductsOfInertiaUnits=kg*mm^2  BasedOnType=DensityFromFile  Density=1000  DensityUnits=kg/m^3  DoExposeReferenceFrame=on  SerializedFrames=<Frames/>  GraphicType=FromGeometry  MarkerShape=Sphere  MarkerSize=10  GraphicVisPropType=SimpleVisualProperties  GraphicDiffuseColor=[1.0 0.0 0.2]  GraphicSpecularColor=[0.5 0.5 0.5 1.0]  GraphicAmbientColor=[0.15 0.15 0.15 1.0]  GraphicEmissiveColor=[0.0 0.0 0.0 1.0]  GraphicShininess=75  GraphicOpacity=smiData.Solid(4).opacity
  Transform : sm_lib/Frames and Transforms/Rigid Transform  TranslationMethod=Cartesian  TranslationStandardOffset=0  TranslationStandardOffsetUnits=m  TranslationStandardAxis=+Z  TranslationCartesianOffset=smiData.RigidTransform(1).translation  TranslationCartesianOffsetUnits=mm  TranslationROffset=0  TranslationROffsetUnits=m  TranslationZOffset=0  TranslationZOffsetUnits=m  TranslationThetaOffset=0  TranslationThetaOffsetUnits=deg  RotationMethod=ArbitraryAxis  RotationAngleUnits=rad  RotationStandardAxis=+Z  RotationAngle=smiData.RigidTransform(1).angle  RotationArbitraryAxis=smiData.RigidTransform(1).axis  FollAlignAxisA=+X  BaseAlignAxisA=+Y  FollAlignAxisB=+Y  BaseAlignAxisB=+Z  RotationSequenceAxes=FollowerAxes  RotationSequence=XYX  RotationSequenceAngles=[0 0 0]  RotationSequenceAnglesUnits=deg  RotationMatrix=[1 0 0; 0 1 0; 0 0 1]  Quaternion=[1 0 0 0]
  Transform1 : sm_lib/Frames and Transforms/Rigid Transform  TranslationMethod=Cartesian  TranslationStandardOffset=0  TranslationStandardOffsetUnits=m  TranslationStandardAxis=+Z  TranslationCartesianOffset=smiData.RigidTransform(10).translation  TranslationCartesianOffsetUnits=mm  TranslationROffset=0  TranslationROffsetUnits=m  TranslationZOffset=0  TranslationZOffsetUnits=m  TranslationThetaOffset=0  TranslationThetaOffsetUnits=deg  RotationMethod=ArbitraryAxis  RotationAngleUnits=rad  RotationStandardAxis=+Z  RotationAngle=smiData.RigidTransform(10).angle  RotationArbitraryAxis=smiData.RigidTransform(10).axis  FollAlignAxisA=+X  BaseAlignAxisA=+Y  FollAlignAxisB=+Y  BaseAlignAxisB=+Z  RotationSequenceAxes=FollowerAxes  RotationSequence=XYX  RotationSequenceAngles=[0 0 0]  RotationSequenceAnglesUnits=deg  RotationMatrix=[1 0 0; 0 1 0; 0 0 1]  Quaternion=[1 0 0 0]
  F1 : PMIOPort  Side=Left
  F : PMIOPort  Port=2  Side=Right
  connections:
  Transform1/RConn1 -- F1/RConn1
  Transform/RConn1 -- F/RConn1
  Transform1/LConn1 -- Transform/LConn1 -- ReferenceFrame/RConn1 -- Solid/RConn1

== system BalanceSimulink/Plant/QUBE Servo 2/Pendulum + Pivot/Pendulum ==
  ReferenceFrame : sm_lib/Frames and Transforms/Reference Frame
  Solid : sm_lib/Body Elements/File Solid  ExtGeomFileName=Pendulum_Default_sldprt.STEP  UnitType=FromFile  ExtGeomFileUnits=m  StepReaderType=HEX  ExportConvexHullGeometry=off  InertiaType=Custom  Mass=smiData.Solid(2).mass  MassUnits=kg  CenterOfMass=smiData.Solid(2).CoM  CenterOfMassUnits=mm  MomentsOfInertia=smiData.Solid(2).MoI  MomentsOfInertiaUnits=kg*mm^2  ProductsOfInertia=smiData.Solid(2).PoI  ProductsOfInertiaUnits=kg*mm^2  BasedOnType=DensityFromFile  Density=1000  DensityUnits=kg/m^3  DoExposeReferenceFrame=on  SerializedFrames=<Frames/>  GraphicType=FromGeometry  MarkerShape=Sphere  MarkerSize=10  GraphicVisPropType=SimpleVisualProperties  GraphicDiffuseColor=[1.0 0.0 0.0]  GraphicSpecularColor=[0.5 0.5 0.5 1.0]  GraphicAmbientColor=[0.15 0.15 0.15 1.0]  GraphicEmissiveColor=[0.0 0.0 0.0 1.0]  GraphicShininess=75  GraphicOpacity=smiData.Solid(2).opacity
  Transform : sm_lib/Frames and Transforms/Rigid Transform  TranslationMethod=Cartesian  TranslationStandardOffset=0  TranslationStandardOffsetUnits=m  TranslationStandardAxis=+Z  TranslationCartesianOffset=smiData.RigidTransform(3).translation  TranslationCartesianOffsetUnits=mm  TranslationROffset=0  TranslationROffsetUnits=m  TranslationZOffset=0  TranslationZOffsetUnits=m  TranslationThetaOffset=0  TranslationThetaOffsetUnits=deg  RotationMethod=ArbitraryAxis  RotationAngleUnits=rad  RotationStandardAxis=+Z  RotationAngle=smiData.RigidTransform(3).angle  RotationArbitraryAxis=smiData.RigidTransform(3).axis  FollAlignAxisA=+X  BaseAlignAxisA=+Y  FollAlignAxisB=+Y  BaseAlignAxisB=+Z  RotationSequenceAxes=FollowerAxes  RotationSequence=XYX  RotationSequenceAngles=[0 0 0]  RotationSequenceAnglesUnits=deg  RotationMatrix=[1 0 0; 0 1 0; 0 0 1]  Quaternion=[1 0 0 0]
  F : PMIOPort  Side=Left
  connections:
  Transform/RConn1 -- F/RConn1
  Transform/LConn1 -- ReferenceFrame/RConn1 -- Solid/RConn1

== system BalanceSimulink/Plant/QUBE Servo 2/Pendulum + Pivot/Pivot ==
  ReferenceFrame : sm_lib/Frames and Transforms/Reference Frame
  Solid : sm_lib/Body Elements/File Solid  ExtGeomFileName=Pivot_Default_sldprt.STEP  UnitType=FromFile  ExtGeomFileUnits=m  StepReaderType=HEX  ExportConvexHullGeometry=off  InertiaType=Custom  Mass=smiData.Solid(3).mass  MassUnits=kg  CenterOfMass=smiData.Solid(3).CoM  CenterOfMassUnits=mm  MomentsOfInertia=smiData.Solid(3).MoI  MomentsOfInertiaUnits=kg*mm^2  ProductsOfInertia=smiData.Solid(3).PoI  ProductsOfInertiaUnits=kg*mm^2  BasedOnType=DensityFromFile  Density=1000  DensityUnits=kg/m^3  DoExposeReferenceFrame=on  SerializedFrames=<Frames/>  GraphicType=FromGeometry  MarkerShape=Sphere  MarkerSize=10  GraphicVisPropType=SimpleVisualProperties  GraphicDiffuseColor=[1.0 1.0 1.0]  GraphicSpecularColor=[0.5 0.5 0.5 1.0]  GraphicAmbientColor=[0.15 0.15 0.15 1.0]  GraphicEmissiveColor=[0.0 0.0 0.0 1.0]  GraphicShininess=75  GraphicOpacity=smiData.Solid(3).opacity
  Transform : sm_lib/Frames and Transforms/Rigid Transform  TranslationMethod=Cartesian  TranslationStandardOffset=0  TranslationStandardOffsetUnits=m  TranslationStandardAxis=+Z  TranslationCartesianOffset=smiData.RigidTransform(2).translation  TranslationCartesianOffsetUnits=mm  TranslationROffset=0  TranslationROffsetUnits=m  TranslationZOffset=0  TranslationZOffsetUnits=m  TranslationThetaOffset=0  TranslationThetaOffsetUnits=deg  RotationMethod=ArbitraryAxis  RotationAngleUnits=rad  RotationStandardAxis=+Z  RotationAngle=smiData.RigidTransform(2).angle  RotationArbitraryAxis=smiData.RigidTransform(2).axis  FollAlignAxisA=+X  BaseAlignAxisA=+Y  FollAlignAxisB=+Y  BaseAlignAxisB=+Z  RotationSequenceAxes=FollowerAxes  RotationSequence=XYX  RotationSequenceAngles=[0 0 0]  RotationSequenceAnglesUnits=deg  RotationMatrix=[1 0 0; 0 1 0; 0 0 1]  Quaternion=[1 0 0 0]
  Transform1 : sm_lib/Frames and Transforms/Rigid Transform  TranslationMethod=Cartesian  TranslationStandardOffset=0  TranslationStandardOffsetUnits=m  TranslationStandardAxis=+Z  TranslationCartesianOffset=smiData.RigidTransform(4).translation  TranslationCartesianOffsetUnits=mm  TranslationROffset=0  TranslationROffsetUnits=m  TranslationZOffset=0  TranslationZOffsetUnits=m  TranslationThetaOffset=0  TranslationThetaOffsetUnits=deg  RotationMethod=ArbitraryAxis  RotationAngleUnits=rad  RotationStandardAxis=+Z  RotationAngle=smiData.RigidTransform(4).angle  RotationArbitraryAxis=smiData.RigidTransform(4).axis  FollAlignAxisA=+X  BaseAlignAxisA=+Y  FollAlignAxisB=+Y  BaseAlignAxisB=+Z  RotationSequenceAxes=FollowerAxes  RotationSequence=XYX  RotationSequenceAngles=[0 0 0]  RotationSequenceAnglesUnits=deg  RotationMatrix=[1 0 0; 0 1 0; 0 0 1]  Quaternion=[1 0 0 0]
  Transform2 : sm_lib/Frames and Transforms/Rigid Transform  TranslationMethod=None  TranslationStandardOffset=0  TranslationStandardOffsetUnits=m  TranslationStandardAxis=+Z  TranslationCartesianOffset=smiData.RigidTransform(4).translation  TranslationCartesianOffsetUnits=mm  TranslationROffset=0  TranslationROffsetUnits=m  TranslationZOffset=0  TranslationZOffsetUnits=m  TranslationThetaOffset=0  TranslationThetaOffsetUnits=deg  RotationMethod=StandardAxis  RotationAngleUnits=deg  RotationStandardAxis=+Z  RotationAngle=-135  RotationArbitraryAxis=smiData.RigidTransform(4).axis  FollAlignAxisA=+X  BaseAlignAxisA=+Y  FollAlignAxisB=+Y  BaseAlignAxisB=+Z  RotationSequenceAxes=FollowerAxes  RotationSequence=XYX  RotationSequenceAngles=[0 0 0]  RotationSequenceAnglesUnits=deg  RotationMatrix=[1 0 0; 0 1 0; 0 0 1]  Quaternion=[1 0 0 0]
  F1 : PMIOPort  Side=Left
  F : PMIOPort  Port=2  Side=Left
  connections:
  Transform2/RConn1 -- F1/RConn1
  Transform1/RConn1 -- Transform2/LConn1
  Transform/RConn1 -- F/RConn1
  Transform1/LConn1 -- Transform/LConn1 -- ReferenceFrame/RConn1 -- Solid/RConn1

== matlab function BalanceSimulink/MATLAB Function ==
  data: obs input; y output
function y = calculatePolicySwingUp(obs)
%#codegen 
    y = get_action_su(obs);
end
